simulink library "MagnTorque"  (R2014b)
settings: Solver=ode45  StartTime=0.0  StopTime=10.0  RelTol=1e-3
undefined symbols (not defined in the file): ConfParam
settings Model: Creator=Hp  LastModifiedBy=Hp

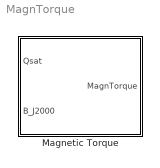
== system MagnTorque ==
  Magnetic Torque : Subsystem

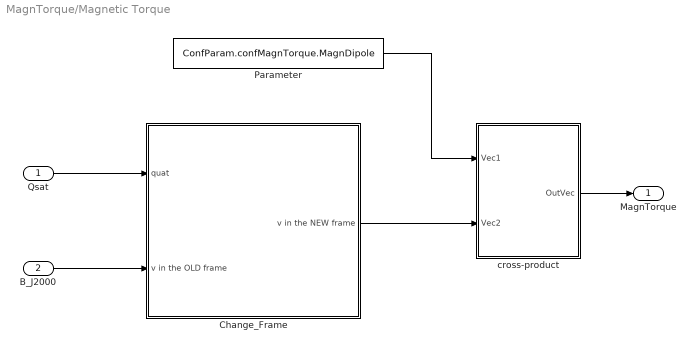
== system MagnTorque/Magnetic Torque ==
  Qsat : Inport
  B_J2000 : Inport  Port=2
  Change_Frame : Subsystem
  Parameter : Constant  Value=ConfParam.confMagnTorque.MagnDipole
  cross-product : Subsystem
  MagnTorque : Outport
  wires:
  B_J2000/1 -> Change_Frame/2(v in the OLD frame)
  Qsat/1 -> Change_Frame/1(quat)
  Change_Frame/1(v in the NEW frame) -> cross-product/2(Vec2)
  cross-product/1(OutVec) -> MagnTorque/1
  Parameter/1 -> cross-product/1(Vec1)

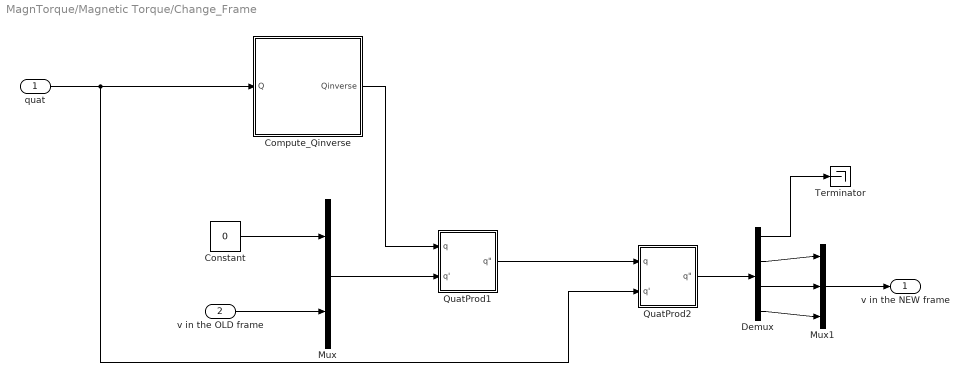
== system MagnTorque/Magnetic Torque/Change_Frame ==
  quat : Inport
  v in the OLD frame : Inport  Port=2
  Compute_Qinverse : Subsystem
  Constant : Constant  Value=0
  Demux : Demux
  Mux : Mux  Inputs=2
  Mux1 : Mux  Inputs=3
  QuatProd1 : Subsystem  TreatAsAtomicUnit=on
      settings: RTWFcnNameOpts=Use subsystem name  RTWFileNameOpts=Use subsystem name
  QuatProd2 : Subsystem  TreatAsAtomicUnit=on
      settings: RTWFcnNameOpts=Use subsystem name  RTWFileNameOpts=Use subsystem name
  Terminator : Terminator
  v in the NEW frame : Outport
  wires:
  QuatProd2/1("q\"") -> Demux/1
  QuatProd1/1("q\"") -> QuatProd2/1(q)
  Demux/4 -> Mux1/3
  Demux/3 -> Mux1/2
  Demux/2 -> Mux1/1
  Mux1/1 -> v in the NEW frame/1
  Compute_Qinverse/1(Qinverse) -> QuatProd1/1(q)
  Constant/1 -> Mux/1
  Mux/1 -> QuatProd1/2(q')
  v in the OLD frame/1 -> Mux/2
  Demux/1 -> Terminator/1
  quat/1 -> Compute_Qinverse/1(Q), QuatProd2/2(q')

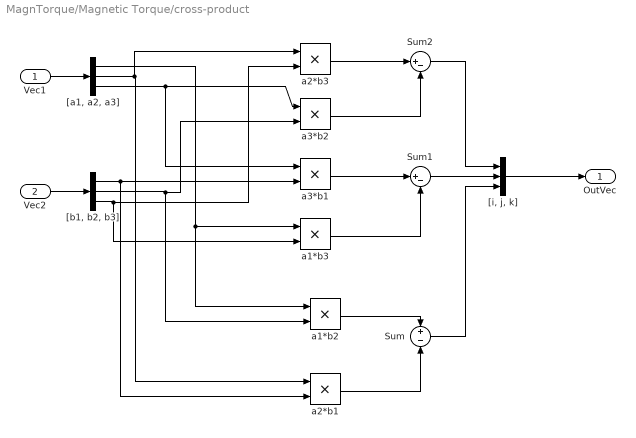
== system MagnTorque/Magnetic Torque/cross-product ==
  Vec1 : Inport
  Vec2 : Inport  Port=2
  Sum : Sum  Inputs=+-
  Sum1 : Sum  Inputs=|+-
  Sum2 : Sum  Inputs=|+-
  "[a1, a2, a3]" : Demux  Outputs=3
  "[b1, b2, b3]" : Demux  Outputs=3
  "[i, j, k]" : Mux  Inputs=3
  a1*b2 : Product
  a1*b3 : Product
  a2*b1 : Product
  a2*b3 : Product
  a3*b1 : Product
  a3*b2 : Product
  OutVec : Outport
  wires:
  a2*b1/1 -> Sum/2
  "[b1, b2, b3]"/1 -> a3*b1/2, a2*b1/2
  "[a1, a2, a3]"/2 -> a2*b3/1, a2*b1/1
  Vec2/1 -> "[b1, b2, b3]"/1
  "[a1, a2, a3]"/1 -> a1*b3/1, a1*b2/1
  Vec1/1 -> "[a1, a2, a3]"/1
  "[b1, b2, b3]"/2 -> a3*b2/2, a1*b2/2
  a1*b2/1 -> Sum/1
  a3*b1/1 -> Sum1/1
  "[a1, a2, a3]"/3 -> a3*b1/1, a3*b2/1
  a2*b3/1 -> Sum2/1
  "[b1, b2, b3]"/3 -> a2*b3/2, a1*b3/2
  a1*b3/1 -> Sum1/2
  "[i, j, k]"/1 -> OutVec/1
  a3*b2/1 -> Sum2/2
  Sum/1 -> "[i, j, k]"/3
  Sum2/1 -> "[i, j, k]"/1
  Sum1/1 -> "[i, j, k]"/2

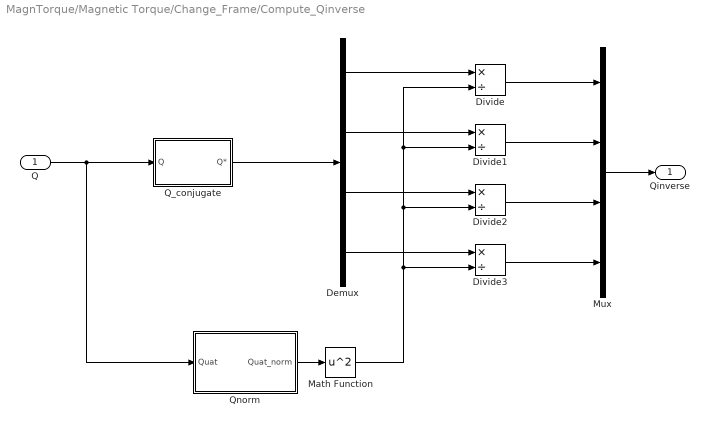
== system MagnTorque/Magnetic Torque/Change_Frame/Compute_Qinverse ==
  Q : Inport
  Demux : Demux
  Divide{,1..3} (4 alike) : Product  Inputs=*/
  Math Function : Math  Operator=square  SaturateOnIntegerOverflow=on
  Mux : Mux
  Q_conjugate : Subsystem
  Qnorm : Subsystem
  Qinverse : Outport
  wires:
  Math Function/1 -> Divide3/2, Divide2/2, Divide1/2, Divide/2
  Demux/3 -> Divide2/1
  Demux/1 -> Divide/1
  Qnorm/1(Quat_norm) -> Math Function/1
  Demux/4 -> Divide3/1
  Q/1 -> Qnorm/1(Quat), Q_conjugate/1(Q)
  Divide3/1 -> Mux/4
  Divide1/1 -> Mux/2
  Divide/1 -> Mux/1
  Q_conjugate/1(Q*) -> Demux/1
  Divide2/1 -> Mux/3
  Demux/2 -> Divide1/1
  Mux/1 -> Qinverse/1

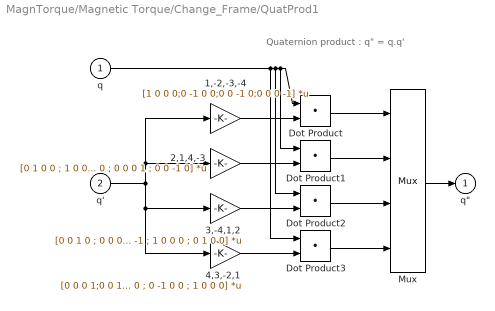
== system MagnTorque/Magnetic Torque/Change_Frame/QuatProd1 ==
  note: Quaternion product : q" = q.q'
  q : Inport  OutDataTypeStr=double  PortDimensions=4
  q' : Inport  Port=2  OutDataTypeStr=double  PortDimensions=4
  1,-2,-3,-4 : Gain  Gain=[1 0 0 0;0 -1 0 0;0 0 -1 0;0 0 0 -1]  Multiplication=Matrix(K*u) (u vector)  SaturateOnIntegerOverflow=on  OutDataTypeStr=Inherit: Same as input  ParamDataTypeStr=Inherit: Same as input
  2,1,4,-3 : Gain  Gain=[0 1 0 0 ; 1 0 0 0 ; 0 0 0 1 ; 0 0 -1 0]  Multiplication=Matrix(K*u) (u vector)  SaturateOnIntegerOverflow=on  OutDataTypeStr=Inherit: Same as input  ParamDataTypeStr=Inherit: Same as input
  3,-4,1,2 : Gain  Gain=[0 0 1 0 ; 0 0 0 -1 ; 1 0 0 0 ; 0 1 0 0]  Multiplication=Matrix(K*u) (u vector)  SaturateOnIntegerOverflow=on  OutDataTypeStr=Inherit: Same as input  ParamDataTypeStr=Inherit: Same as input
  4,3,-2,1 : Gain  Gain=[0 0 0 1;0 0 1 0 ; 0 -1 0 0 ; 1 0 0 0]  Multiplication=Matrix(K*u) (u vector)  SaturateOnIntegerOverflow=on  OutDataTypeStr=Inherit: Same as input  ParamDataTypeStr=Inherit: Same as input
  Dot Product{,1..3} (4 alike) : DotProduct  InputSameDT=on  OutDataTypeStr=Inherit: Inherit via internal rule
  Mux : Mux
  "q\"" : Outport  OutDataTypeStr=double  PortDimensions=4  InitialOutput=0
  wires:
  Mux/1 -> "q\""/1
  Dot Product3/1 -> Mux/4
  Dot Product2/1 -> Mux/3
  Dot Product1/1 -> Mux/2
  Dot Product/1 -> Mux/1
  q/1 -> Dot Product3/1, Dot Product2/1, Dot Product1/1, Dot Product/1
  4,3,-2,1/1 -> Dot Product3/2
  3,-4,1,2/1 -> Dot Product2/2
  2,1,4,-3/1 -> Dot Product1/2
  1,-2,-3,-4/1 -> Dot Product/2
  q'/1 -> 2,1,4,-3/1, 1,-2,-3,-4/1, 4,3,-2,1/1, 3,-4,1,2/1

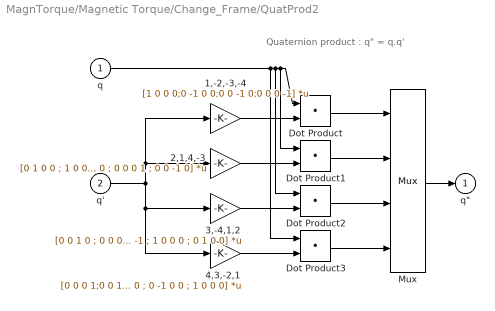
== system MagnTorque/Magnetic Torque/Change_Frame/QuatProd2 ==
  note: Quaternion product : q" = q.q'
  q : Inport  OutDataTypeStr=double  PortDimensions=4
  q' : Inport  Port=2  OutDataTypeStr=double  PortDimensions=4
  1,-2,-3,-4 : Gain  Gain=[1 0 0 0;0 -1 0 0;0 0 -1 0;0 0 0 -1]  Multiplication=Matrix(K*u) (u vector)  SaturateOnIntegerOverflow=on  OutDataTypeStr=Inherit: Same as input  ParamDataTypeStr=Inherit: Same as input
  2,1,4,-3 : Gain  Gain=[0 1 0 0 ; 1 0 0 0 ; 0 0 0 1 ; 0 0 -1 0]  Multiplication=Matrix(K*u) (u vector)  SaturateOnIntegerOverflow=on  OutDataTypeStr=Inherit: Same as input  ParamDataTypeStr=Inherit: Same as input
  3,-4,1,2 : Gain  Gain=[0 0 1 0 ; 0 0 0 -1 ; 1 0 0 0 ; 0 1 0 0]  Multiplication=Matrix(K*u) (u vector)  SaturateOnIntegerOverflow=on  OutDataTypeStr=Inherit: Same as input  ParamDataTypeStr=Inherit: Same as input
  4,3,-2,1 : Gain  Gain=[0 0 0 1;0 0 1 0 ; 0 -1 0 0 ; 1 0 0 0]  Multiplication=Matrix(K*u) (u vector)  SaturateOnIntegerOverflow=on  OutDataTypeStr=Inherit: Same as input  ParamDataTypeStr=Inherit: Same as input
  Dot Product{,1..3} (4 alike) : DotProduct  InputSameDT=on  OutDataTypeStr=Inherit: Inherit via internal rule
  Mux : Mux
  "q\"" : Outport  OutDataTypeStr=double  PortDimensions=4  InitialOutput=0
  wires:
  Mux/1 -> "q\""/1
  Dot Product3/1 -> Mux/4
  Dot Product2/1 -> Mux/3
  Dot Product1/1 -> Mux/2
  Dot Product/1 -> Mux/1
  q/1 -> Dot Product3/1, Dot Product2/1, Dot Product1/1, Dot Product/1
  4,3,-2,1/1 -> Dot Product3/2
  3,-4,1,2/1 -> Dot Product2/2
  2,1,4,-3/1 -> Dot Product1/2
  1,-2,-3,-4/1 -> Dot Product/2
  q'/1 -> 2,1,4,-3/1, 1,-2,-3,-4/1, 4,3,-2,1/1, 3,-4,1,2/1

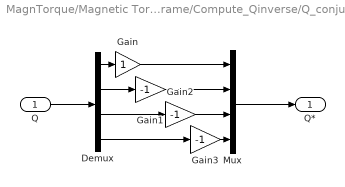
== system MagnTorque/Magnetic Torque/Change_Frame/Compute_Qinverse/Q_conjugate ==
  Q : Inport
  Demux : Demux
  Gain : Gain
  Gain1 : Gain  Gain=-1
  Gain2 : Gain  Gain=-1
  Gain3 : Gain  Gain=-1
  Mux : Mux
  Q* : Outport
  wires:
  Demux/1 -> Gain/1
  Gain/1 -> Mux/1
  Mux/1 -> Q*/1
  Demux/4 -> Gain3/1
  Gain1/1 -> Mux/2
  Demux/3 -> Gain2/1
  Demux/2 -> Gain1/1
  Gain2/1 -> Mux/3
  Q/1 -> Demux/1
  Gain3/1 -> Mux/4

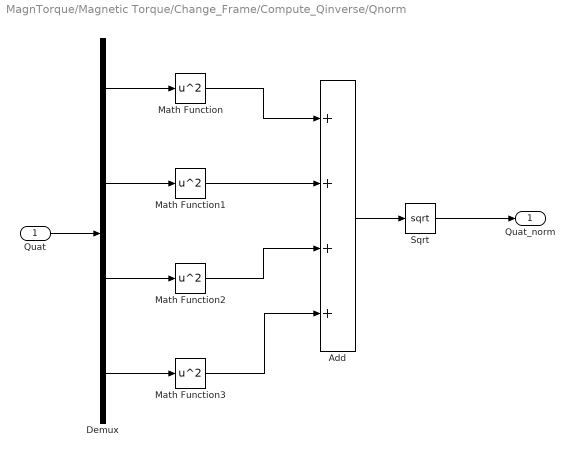
== system MagnTorque/Magnetic Torque/Change_Frame/Compute_Qinverse/Qnorm ==
  Quat : Inport
  Add : Sum  Inputs=++++
  Demux : Demux
  Math Function{,1..3} (4 alike) : Math  Operator=square  SaturateOnIntegerOverflow=on
  Sqrt : Sqrt  SaturateOnIntegerOverflow=on
  Quat_norm : Outport
  wires:
  Math Function2/1 -> Add/3
  Math Function/1 -> Add/1
  Add/1 -> Sqrt/1
  Math Function3/1 -> Add/4
  Math Function1/1 -> Add/2
  Demux/3 -> Math Function2/1
  Demux/1 -> Math Function/1
  Demux/4 -> Math Function3/1
  Sqrt/1 -> Quat_norm/1
  Demux/2 -> Math Function1/1
  Quat/1 -> Demux/1
